simulink model "lungs_test"  (R2026a)
settings: Solver=ode15s
libraries: scuba_lib x2, nesl_utility x2, fl_lib x2
settings Model: Creator=grouleau  LastModifiedBy=grouleau

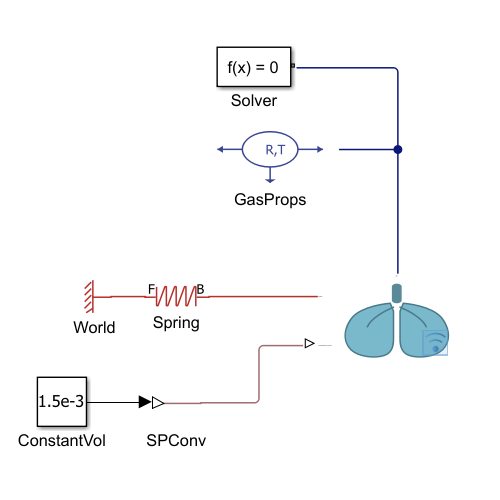
[thumbnail: Simulink's stored preview of the top-level diagram]
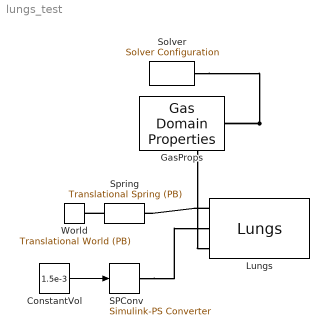
== system lungs_test ==
  ConstantVol : Constant  Value=1.5e-3
  GasProps : scuba_lib/gas/elements/Gas Domain Properties  R_gas=8.314 J/(K*mol)  T=293.15 K  n_dot_thru_specify=off  n_dot_thru_priority=None  n_dot_thru=0 mol/s  n_dot_thru_nominal_specify=off  n_dot_thru_nominal_value=1  n_dot_thru_nominal_unit=mol/s
  Lungs : scuba_lib/gas/elements/Lungs  n_init=0.104 mol  rho_water=1025 kg/m^3  P_atm=101325 Pa  n_dot_specify=off  n_dot_priority=None  n_dot=0 mol/s  n_dot_nominal_specify=off  n_dot_nominal_value=1  n_dot_nominal_unit=mol/s  f_specify=off  f_priority=None  f=0 N  f_nominal_specify=off  f_nominal_value=1  f_nominal_unit=N  P_lung_specify=off  P_lung_priority=None  P_lung=101325 Pa  P_lung_nominal_specify=off  P_lung_nominal_value=1  P_lung_nominal_unit=Pa
  SPConv : nesl_utility/Simulink-PS Converter  PhysicalDomain=network_engine_domain  SubClassName=ps_input  LeftPortType=input  RightPortType=output  PseudoPeriodic=off  Frequencies=[]  NoiseDistribution=none  NoiseParameters=[]  Unit=1  AffineConversion=off  FilteringAndDerivatives=provide  SimscapeFilterOrder=1  InputFilterTimeConstant=0.001  UdotUserProvided=0
  Solver : nesl_utility/Solver Configuration  PhysicalDomain=network_engine_domain  SubClassName=solver  LeftPortType=input  RightPortType=generic  Tones=[]  Harmonics=[]  SimulateNoise=off  Profile=off  UseLocalSampling=off  EnableSwitchedLinearOptims=on  FrequencyDomain=off  UseCCode=off  RelTol=0.001  AbsTol=0.001  MinStep=1e-09  ToWorkspace=off  RevertToSquareIcSolve=off  NumHomotopyIterations=100  PhasorMode=off  PhasorModeNumHarmonics=1  ConsistencySolver=NEWTON_XTOL_AFTER_FTOL  CanonicalOrdering=CANONICAL  OptimizeIntermediates=OPTIMIZED  IndexReductionMethod=DerivativeReplacement  DoDC=off  ResidualTolerance=1e-09  ConsistencyTolSource=GLOBAL  ConsistencyAbsTol=0.001  ConsistencyRelTol=0.001  ConsistencyTolFactor=0.001  UseLocalSolver=off  LocalSolverChoice=NE_BACKWARD_EULER_ADVANCER  ResolveIndetEquations=on  FunctionEvalNumThread=1  LocalSolverSampleTime=0.001  DoFixedCost=off  MaxNonlinIter=3  MaxModeIter=2  ComputeImpulses=off  ImpulseIterations=2  LinearAlgebra=auto  LinearAlgebraNumThread=0  EquationFormulation=NE_TIME_EF  DelaysMemoryBudget=1024  AutomaticFiltering=on  FilteringTimeConstant=0.001  PartitionStorageMethod=AS_NEEDED  PartitionMemoryBudget=1024  PartitionMethod=ROBUST  MultibodyUseLocalSolver=off  MultibodyLocalSolverChoice=ODE1  MultibodyLocalSolverSampleTime=0.001
  Spring : fl_lib/Translational/Elements/Translational Spring (PB)  stiffness=1e3 N/m  f_specify=off  f_priority=None  f=0 N  f_nominal_specify=off  f_nominal_value=1  f_nominal_unit=N  deformation_specify=off  deformation_priority=None  deformation=0 m  deformation_nominal_specify=off  deformation_nominal_value=1  deformation_nominal_unit=m  length_specify=off  length_priority=None  length=0.1 m  length_nominal_specify=off  length_nominal_value=1  length_nominal_unit=m  rest_length_specify=off  rest_length_priority=None  rest_length=0.1 m  rest_length_nominal_specify=off  rest_length_nominal_value=1  rest_length_nominal_unit=m
  World : fl_lib/Translational/Elements/Translational World (PB)
  wires:
  ConstantVol/1 -> SPConv/1
  connections:
  SPConv/RConn1 -- Lungs/LConn2
  GasProps/LConn1 -- Solver/RConn1 -- Lungs/LConn3
  Lungs/LConn1 -- Spring/LConn1
  Spring/RConn1 -- World/RConn1
